simulink model "task3"  (Simulink 7.5)
settings: Solver=ode3  StartTime=0.0  StopTime=10.0  RelTol=1e-3
settings Model: Creator=Dranik_win  LastModifiedBy=Dranik_win
settings SimEventsCC: propDiagAttribOutput=1  propDiagFcnCallOutput=1  propDiagStatOutput=0

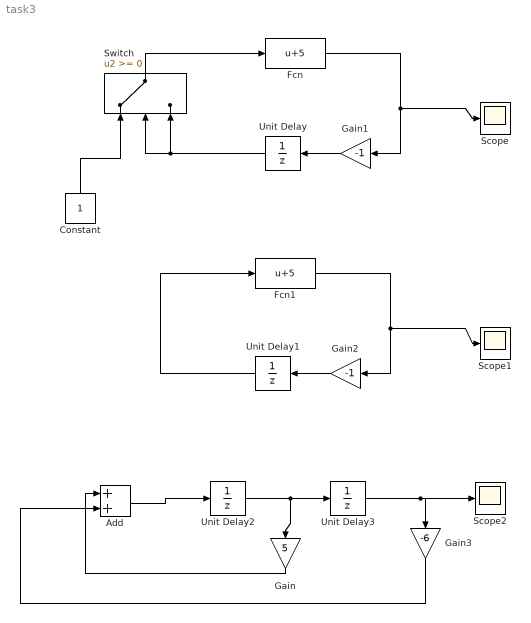
== system task3 ==
  Add : Sum  OutDataType=fixdt(1, 16)  OutScaling=2^-10
  Constant : Constant  OutDataType=fixdt(1, 16)  OutScaling=2^0
  Fcn : Fcn  Expr=u+5  SampleTime=1
  Fcn1 : Fcn  Expr=u+5  SampleTime=1
  Gain : Gain  Gain=5  ParameterDataType=fixdt(1, 16)  ParameterScaling=2^0  OutDataType=fixdt(1, 16)  OutScaling=2^0
  Gain1 : Gain  Gain=-1  ParameterDataType=fixdt(1, 16)  ParameterScaling=2^0  OutDataType=fixdt(1, 16)  OutScaling=2^0
  Gain2 : Gain  Gain=-1  ParameterDataType=fixdt(1, 16)  ParameterScaling=2^0  OutDataType=fixdt(1, 16)  OutScaling=2^0
  Gain3 : Gain  Gain=-6  ParameterDataType=fixdt(1, 16)  ParameterScaling=2^0  OutDataType=fixdt(1, 16)  OutScaling=2^0
  Scope : Scope
      settings: YMin=-2  YMax=7
  Scope1 : Scope
      settings: YMin=-2  YMax=7
  Scope2 : Scope
      settings: YMin=-2  YMax=7  SaveName=ScopeData2
  Switch : Switch  OutDataType=fixdt(1, 16)  OutScaling=2^0
  Unit Delay : UnitDelay  SampleTime=-1
  Unit Delay1 : UnitDelay  X0=1  SampleTime=-1
  Unit Delay2 : UnitDelay  X0=1  SampleTime=-1
  Unit Delay3 : UnitDelay  X0=1  SampleTime=-1
  wires:
  Fcn/1 -> Gain1/1, Scope/1
  Gain1/1 -> Unit Delay/1
  Unit Delay/1 -> Switch/2, Switch/3
  Switch/1 -> Fcn/1
  Constant/1 -> Switch/1
  Fcn1/1 -> Gain2/1, Scope1/1
  Gain2/1 -> Unit Delay1/1
  Unit Delay1/1 -> Fcn1/1
  Unit Delay2/1 -> Unit Delay3/1, Gain/1
  Unit Delay3/1 -> Gain3/1, Scope2/1
  Add/1 -> Unit Delay2/1
  Gain/1 -> Add/1
  Gain3/1 -> Add/2
